simulink model "untitled"  (R2023b)
settings: Solver=VariableStepAuto  StartTime=0.0  StopTime=10.0  RelTol=1e-3
undefined symbols (not defined in the file or in its folder): A_sn, B_sn, C_sn, D_sn, E_sn, F_sn, G_sn, H_sn
settings Model: Creator=henriquesaito  LastModifiedBy=henriquesaito

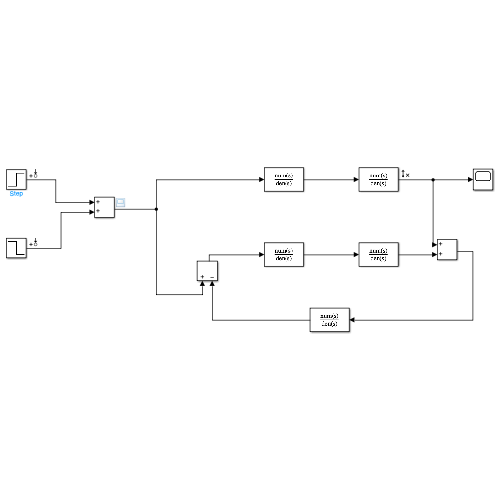
[thumbnail: Simulink's stored preview of the top-level diagram]
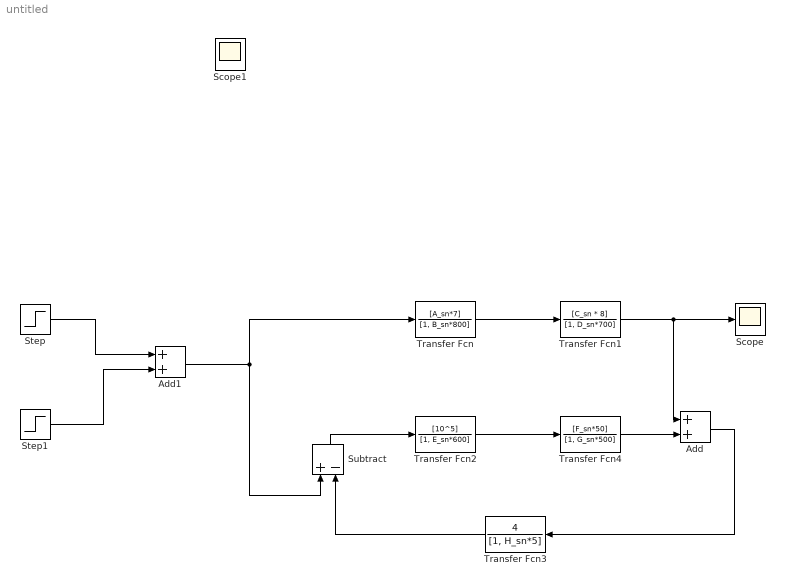
== system untitled ==
  Add : Sum
  Add1 : Sum
  Scope : Scope
  Step : Step  Time=0.025  SampleTime=0
  Step1 : Step  Time=0.050  After=-1  SampleTime=0
  Subtract : Sum  Inputs=+-
  Transfer Fcn : TransferFcn  Numerator=[A_sn*7]  Denominator=[1, B_sn*800]
  Transfer Fcn1 : TransferFcn  Numerator=[C_sn * 8]  Denominator=[1, D_sn*700]
  Transfer Fcn2 : TransferFcn  Numerator=[10^5]  Denominator=[1, E_sn*600]
  Transfer Fcn3 : TransferFcn  Numerator=[4]  Denominator=[1, H_sn*5]
  Transfer Fcn4 : TransferFcn  Numerator=[F_sn*50]  Denominator=[1, G_sn*500]
  Scope1 : Scope
  wires:
  Transfer Fcn/1 -> Transfer Fcn1/1
  Transfer Fcn1/1 -> Add/1, Scope/1
  Transfer Fcn4/1 -> Add/2
  Add/1 -> Transfer Fcn3/1
  Transfer Fcn3/1 -> Subtract/2
  Subtract/1 -> Transfer Fcn2/1
  Transfer Fcn2/1 -> Transfer Fcn4/1
  Add1/1 -> Transfer Fcn/1, Subtract/1
  Step1/1 -> Add1/2
  Step/1 -> Add1/1
